simulink model "kalman"  (R2015b)
settings: Solver=ode4  SolverMode=SingleTasking  StartTime=0.0  StopTime=SIM_TIME  FixedStep=STEP_TIME  RelTol=1e-3
values from neighbouring files (symbols this model uses):
  A = zeros(4)    [kalman.m]
  B = zeros(4,1)    [kalman.m]
  Bv = zeros(4,2)    [kalman.m]
  C = zeros(2,4)    [kalman.m]
  F = systemus_d.a    [kalman.m]
  G = systemus_d.b(:,size(B,2))    [kalman.m]
  SEED_VEC_v1 = [1 2]    [kalman.m]
  SEED_VEC_v2 = [3 4]    [kalman.m]
  sys_init = [0 0 0 0]    [kalman.m]
  T_c = STEP_TIME    (= 0.0001)    [kalman.m]
  T_s = 1    [kalman.m]
  v1_switch = 1    [kalman.m]
  v2_switch = 1    [kalman.m]
undefined symbols (not defined in the file or in its folder): L
libraries: simulink x2
settings Model: Creator=s134082  LastModifiedBy=s134082

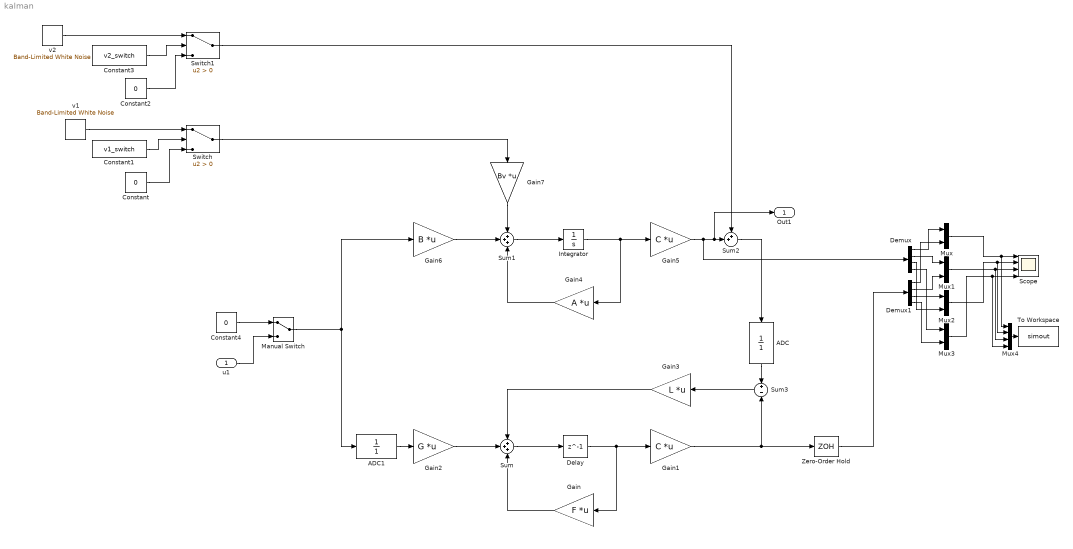
== system kalman ==
  u1 : Inport
  ADC : DiscreteTransferFcn  Denominator=[1]  SampleTime=T_s
  ADC1 : DiscreteTransferFcn  Denominator=[1]  SampleTime=T_s
  Constant : Constant  Value=0
  Constant1 : Constant  Value=v1_switch
  Constant2 : Constant  Value=0
  Constant3 : Constant  Value=v2_switch
  Constant4 : Constant  Value=0
  Delay : Delay  DelayLength=1  InitialCondition=0  SampleTime=T_s
  Demux : Demux
  Demux1 : Demux
  Gain : Gain  Gain=F  Multiplication=Matrix(K*u)
  Gain1 : Gain  Gain=C  Multiplication=Matrix(K*u)
  Gain2 : Gain  Gain=G  Multiplication=Matrix(K*u)
  Gain3 : Gain  Gain=L  Multiplication=Matrix(K*u)
  Gain4 : Gain  Gain=A  Multiplication=Matrix(K*u)
  Gain5 : Gain  Gain=C  Multiplication=Matrix(K*u)
  Gain6 : Gain  Gain=B  Multiplication=Matrix(K*u)
  Gain7 : Gain  Gain=Bv  Multiplication=Matrix(K*u)
  Integrator : Integrator  Priority=1  InitialCondition=sys_init
  Manual Switch : ManualSwitch
  Mux{,1..3} (4 alike) : Mux  Inputs=2
  Mux4 : Mux
  Scope : Scope  NumInputPorts=4
  Sum : Sum  Inputs=+++
  Sum1 : Sum  Inputs=+++
  Sum2 : Sum  Inputs=++|
  Sum3 : Sum  Inputs=+|-
  Switch : Switch  Criteria=u2 > Threshold
  Switch1 : Switch  Criteria=u2 > Threshold
  To Workspace : ToWorkspace  VariableName=simout  SaveFormat=Timeseries  SampleTime=-1
  Zero-Order Hold : ZeroOrderHold  SampleTime=T_s
  v1 : simulink/Sources/Band-Limited White Noise  Cov=v1  Ts=T_c  seed=[SEED_VEC_v1]
  v2 : simulink/Sources/Band-Limited White Noise  Cov=v2  Ts=T_c  seed=[SEED_VEC_v2]
  Out1 : Outport
  wires:
  Gain3/1 -> Sum/1
  Gain/1 -> Sum/3
  Gain2/1 -> Sum/2
  Gain7/1 -> Sum1/1
  Gain4/1 -> Sum1/3
  Integrator/1 -> Gain5/1, Gain4/1
  Sum1/1 -> Integrator/1
  Gain6/1 -> Sum1/2
  Gain1/1 -> Zero-Order Hold/1, Sum3/2
  Sum3/1 -> Gain3/1
  v1/1 -> Switch/1
  Constant/1 -> Switch/3
  Constant1/1 -> Switch/2
  v2/1 -> Switch1/1
  Constant3/1 -> Switch1/2
  Constant2/1 -> Switch1/3
  Constant4/1 -> Manual Switch/1
  u1/1 -> Manual Switch/2
  Manual Switch/1 -> Gain6/1, ADC1/1
  Delay/1 -> Gain/1, Gain1/1
  Sum/1 -> Delay/1
  Switch1/1 -> Sum2/1
  Switch/1 -> Gain7/1
  Gain5/1 -> Demux/1, Out1/1, Sum2/2
  Demux/1 -> Mux/1
  Demux1/1 -> Mux/2
  Demux/2 -> Mux1/1
  Demux1/2 -> Mux1/2
  Demux/3 -> Mux2/1
  Demux1/3 -> Mux2/2
  Demux/4 -> Mux3/1
  Demux1/4 -> Mux3/2
  Mux/1 -> Mux4/1, Scope/1
  Mux2/1 -> Mux4/2, Scope/2
  Mux1/1 -> Mux4/3, Scope/3
  Mux3/1 -> Mux4/4, Scope/4
  Mux4/1 -> To Workspace/1
  ADC1/1 -> Gain2/1
  ADC/1 -> Sum3/1
  Sum2/1 -> ADC/1
  Zero-Order Hold/1 -> Demux1/1
